simulink model "DC_motor"  (R2020b)
settings: Solver=ode5  StartTime=0.0  StopTime=1  FixedStep=1e-4  RelTol=1e-3
values from neighbouring files (symbols this model uses):
  Kd = par(bestchrom,3)    [ga_PID_Motor.m]
  Ki = par(bestchrom,2)    [ga_PID_Motor.m]
  Kp = par(bestchrom,1)    [ga_PID_Motor.m]
settings Model: Creator=ACER  LastModifiedBy=ACER

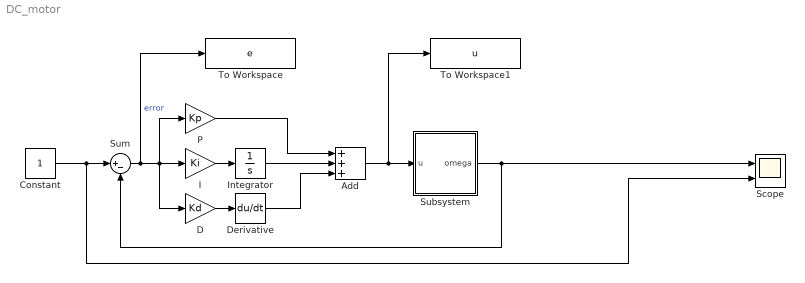
== system DC_motor ==
  Add : Sum  Inputs=+++
  Constant : Constant
  D : Gain  Gain=Kd
  Derivative : Derivative
  I : Gain  Gain=Ki
  Integrator : Integrator
  P : Gain  Gain=Kp
  Scope : Scope  NumInputPorts=2
  Subsystem : Subsystem  mask{Parameter1=0}
      mask prompts: Parameter1 "omega"
  Sum : Sum  Inputs=|+-
  To Workspace : ToWorkspace  VariableName=e  SampleTime=-1
  To Workspace1 : ToWorkspace  VariableName=u  SampleTime=-1
  wires:
  Subsystem/1(omega) -> Sum/2, Scope/1
  Add/1 -> To Workspace1/1, Subsystem/1(u)
  Constant/1 -> Scope/2, Sum/1
  P/1 -> Add/1
  Sum/1 -> To Workspace/1, P/1, D/1, I/1  "error"
  D/1 -> Derivative/1
  Derivative/1 -> Add/3
  I/1 -> Integrator/1
  Integrator/1 -> Add/2

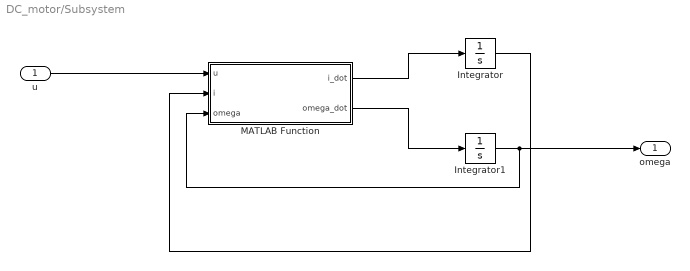
== system DC_motor/Subsystem ==
  u : Inport
  Integrator : Integrator
  Integrator1 : Integrator
  MATLAB Function : MATLAB Function  TreatAsAtomicUnit=on
  omega : Outport
  wires:
  u/1 -> MATLAB Function/1(u)
  Integrator1/1 -> omega/1, MATLAB Function/3(omega)
  MATLAB Function/2(omega_dot) -> Integrator1/1
  MATLAB Function/1(i_dot) -> Integrator/1
  Integrator/1 -> MATLAB Function/2(i)

== matlab function DC_motor/Subsystem/MATLAB Function ==
  data: u input; i input; i_dot output; omega_dot output; omega input
function [i_dot, omega_dot] = fcn(u, i, omega)
R = 1;
L = 0.03;
Km = 0.2;
Kb = 0.2;
J = 0.02;
Kf = 0.2;
i_dot = -R/L*i - Kb/L*omega +1/L*u;
omega_dot = Km/J*i - Kf/J*omega;
